simulink model "mra_2"  (Simulink 7.8)
settings: Solver=ode45  StartTime=0.0  StopTime=10.0  RelTol=1e-3
values from neighbouring files (symbols this model uses):
  g0 = h0    [G722_1.m]    (also in audio_test1.m = gsy(:,1); audio_test2.m = gsy(:,1))
  g1 = fliplr(h1)    [G722_1.m]    (also in audio_test1.m = gsy(:,2); audio_test2.m = gsy(:,2))
  h0 = zeros(1,L)    [G722_1.m]    (also in audio_test1.m = han(:,1); audio_test2.m = han(:,1); band4.m = fir1(nf, 2*ftp))
  h1 = firpm(128,f,m)    [CFIR_1.m]    (also in G722_1.m = (-1).^(0:L-1).*h0; audio_test1.m = han(:,2); audio_test2.m = han(:,2))
  Ts = 1/fs    (= 6.25e-05)    [G722_1.m]    (also in adaptiv_2.m = 0.001; adaptiv_3.m = 0.001; adaptiv_4.m = 0.001; adaptiv_5.m = 0.001)
libraries: dspsigops x16, dsparch4 x2
settings Model: Creator=svenhoffmann  LastModifiedBy=josef  ExtModeAutoUpdateStatusClock=off
settings DataIOCC: SignalLoggingName=sigsOut
settings OptimizationCC: InitFltsAndDblsToZero=on
settings DebuggingCC: SaveWithParameterizedLinksMsg=none  SignalResolutionControl=TryResolveAllWithWarning  SolverPrmCheckMsg=none  MultiTaskDSMMsg=warning  MultiTaskCondExecSysMsg=none  FcnCallInpInsideContextMsg=Use local settings  StrictBusMsg=None
settings HardwareCC: TargetUnknown=on
settings RTWCC: IncludeERTFirstTime=on
settings GRTTargetCC: TargetFcnLib=ansi_tfl_tmw.mat

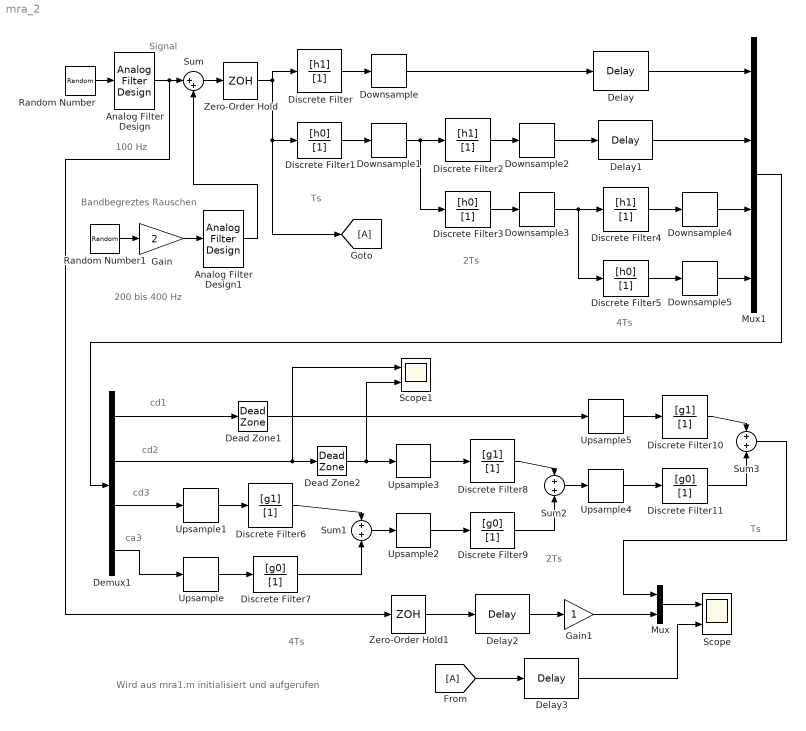
== system mra_2 ==
  note: Ts
  note: 2Ts
  note: 4Ts
  note: 4Ts
  note: 2Ts
  note: Ts
  note: cd1
  note: cd2
  note: cd3
  note: ca3
  note: Signal
  note: Bandbegreztes
      | Rauschen
  note: 200 bis 400 Hz
  note: 100 Hz
  note: Wird aus mra1.m initialisiert und aufgerufen
  Analog Filter Design : dsparch4/Analog Filter Design  method=Butterworth  filttype=Lowpass  N=8  Wlo=2*pi*100  Whi=80  Rp=2  Rs=40
  Analog Filter Design1 : dsparch4/Analog Filter Design  method=Chebyshev I  filttype=Bandpass  N=8  Wlo=2*pi*150  Whi=2*pi*400  Rp=2  Rs=60
  Dead Zone1 : DeadZone  LowerValue=-10  UpperValue=10  SaturateOnIntegerOverflow=on
  Dead Zone2 : DeadZone  LowerValue=-10  UpperValue=10  SaturateOnIntegerOverflow=on
  Delay : dspsigops/Delay  InputProcessing=Inherited (this choice will be removed - see release notes)  dly_unit=Samples  delay=delay2  ic_detail=off  dif_ic_for_ch=off  dif_ic_for_dly=off  ic=0  reset_popup=None
  Delay1 : dspsigops/Delay  InputProcessing=Inherited (this choice will be removed - see release notes)  dly_unit=Samples  delay=delay1  ic_detail=off  dif_ic_for_ch=off  dif_ic_for_dly=off  ic=0  reset_popup=None
  Delay2 : dspsigops/Delay  InputProcessing=Inherited (this choice will be removed - see release notes)  dly_unit=Samples  delay=delay3  ic_detail=off  dif_ic_for_ch=off  dif_ic_for_dly=off  ic=0  reset_popup=None
  Delay3 : dspsigops/Delay  InputProcessing=Inherited (this choice will be removed - see release notes)  dly_unit=Samples  delay=delay3  ic_detail=off  dif_ic_for_ch=off  dif_ic_for_dly=off  ic=0  reset_popup=None
  Demux1 : Demux
  Discrete Filter : DiscreteFilter  Numerator=[h1]  Denominator=[1]  SampleTime=Ts
  Discrete Filter1 : DiscreteFilter  Numerator=[h0]  Denominator=[1]  SampleTime=Ts
  Discrete Filter10 : DiscreteFilter  Numerator=[g1]  Denominator=[1]  SampleTime=Ts
  Discrete Filter11 : DiscreteFilter  Numerator=[g0]  Denominator=[1]  SampleTime=Ts
  Discrete Filter2 : DiscreteFilter  Numerator=[h1]  Denominator=[1]  SampleTime=2*Ts
  Discrete Filter3 : DiscreteFilter  Numerator=[h0]  Denominator=[1]  SampleTime=2*Ts
  Discrete Filter4 : DiscreteFilter  Numerator=[h1]  Denominator=[1]  SampleTime=4*Ts
  Discrete Filter5 : DiscreteFilter  Numerator=[h0]  Denominator=[1]  SampleTime=4*Ts
  Discrete Filter6 : DiscreteFilter  Numerator=[g1]  Denominator=[1]  SampleTime=4*Ts
  Discrete Filter7 : DiscreteFilter  Numerator=[g0]  Denominator=[1]  SampleTime=4*Ts
  Discrete Filter8 : DiscreteFilter  Numerator=[g1]  Denominator=[1]  SampleTime=2*Ts
  Discrete Filter9 : DiscreteFilter  Numerator=[g0]  Denominator=[1]  SampleTime=2*Ts
  Downsample{,1..5} (6 alike) : dspsigops/Downsample  N=2  phase=0  InputProcessing=Inherited (this choice will be removed - see release notes)  RateOptions=Enforce single-rate processing  smode=Allow multirate  fmode=Maintain input frame size  ic=0
  Gain : Gain  Gain=2  SaturateOnIntegerOverflow=on  OutDataTypeStr=Inherit: Same as input  ParamDataTypeStr=Inherit: Same as input
  Gain1 : Gain  SaturateOnIntegerOverflow=on  OutDataTypeStr=Inherit: Same as input  ParamDataTypeStr=Inherit: Same as input
  Mux : Mux  Inputs=2
  Mux1 : Mux
  Random Number : RandomNumber  Seed=123978  SampleTime=0
  Random Number1 : RandomNumber  SampleTime=0
  Scope : Scope  NumInputPorts=2
      settings: YMin=-1~-2  YMax=1~1.75
  Scope1 : Scope  NumInputPorts=2
      settings: YMin=-3~-1  YMax=3~1
  Sum : Sum  Inputs=|++  SaturateOnIntegerOverflow=on
  Sum1 : Sum  Inputs=+|+  SaturateOnIntegerOverflow=on
  Sum2 : Sum  Inputs=+|+  SaturateOnIntegerOverflow=on
  Sum3 : Sum  Inputs=+|+  SaturateOnIntegerOverflow=on
  Upsample{,1..5} (6 alike) : dspsigops/Upsample  N=2  phase=0  InputProcessing=Inherited (this choice will be removed - see release notes)  RateOptions=Allow multirate processing  ic=0  mode=Unused parameter value
  Zero-Order Hold : ZeroOrderHold  SampleTime=Ts
  Zero-Order Hold1 : ZeroOrderHold  SampleTime=Ts
  wires:
  Random Number/1 -> Analog Filter Design/1
  Analog Filter Design/1 -> Zero-Order Hold1/1, Sum/1
  Random Number1/1 -> Gain/1
  Discrete Filter/1 -> Downsample/1
  Discrete Filter1/1 -> Downsample1/1
  Downsample1/1 -> Discrete Filter3/1, Discrete Filter2/1
  Discrete Filter4/1 -> Downsample4/1
  Discrete Filter5/1 -> Downsample5/1
  Downsample3/1 -> Discrete Filter5/1, Discrete Filter4/1
  Sum/1 -> Zero-Order Hold/1
  Discrete Filter2/1 -> Downsample2/1
  Discrete Filter3/1 -> Downsample3/1
  Downsample/1 -> Delay/1
  Downsample2/1 -> Delay1/1
  Downsample5/1 -> Mux1/4
  Downsample4/1 -> Mux1/3
  Delay1/1 -> Mux1/2
  Delay/1 -> Mux1/1
  Mux1/1 -> Demux1/1
  Upsample1/1 -> Discrete Filter6/1
  Upsample/1 -> Discrete Filter7/1
  Discrete Filter6/1 -> Sum1/1
  Discrete Filter7/1 -> Sum1/2
  Sum1/1 -> Upsample2/1
  Upsample2/1 -> Discrete Filter9/1
  Upsample3/1 -> Discrete Filter8/1
  Discrete Filter8/1 -> Sum2/1
  Discrete Filter9/1 -> Sum2/2
  Sum2/1 -> Upsample4/1
  Upsample4/1 -> Discrete Filter11/1
  Upsample5/1 -> Discrete Filter10/1
  Discrete Filter10/1 -> Sum3/1
  Discrete Filter11/1 -> Sum3/2
  Mux/1 -> Scope/1
  Sum3/1 -> Mux/1
  Delay2/1 -> Gain1/1
  Zero-Order Hold/1 -> Discrete Filter/1, Discrete Filter1/1, [A]
  Gain1/1 -> Mux/2
  Dead Zone1/1 -> Upsample5/1
  Dead Zone2/1 -> Upsample3/1, Scope1/2
  Zero-Order Hold1/1 -> Delay2/1
  Gain/1 -> Analog Filter Design1/1
  Analog Filter Design1/1 -> Sum/2
  [A] -> Delay3/1
  Delay3/1 -> Scope/2
  Demux1/1 -> Dead Zone1/1
  Demux1/2 -> Dead Zone2/1, Scope1/1
  Demux1/3 -> Upsample1/1
  Demux1/4 -> Upsample/1
